simulink model "state_feedback_control_4_1_wout_velocity_eqn_2"  (R2018b)
settings: Solver=VariableStepAuto  StartTime=0.0  StopTime=10.0  RelTol=1e-3
values from neighbouring files (symbols this model uses):
  alpha = 10    [in_lab.m]
  f1 = F(1)    [in_lab.m]
  f2 = F(2)    [in_lab.m]
libraries: cstblocks x1
settings Model: Creator=pranshumalik14  LastModifiedBy=pranshumalik14

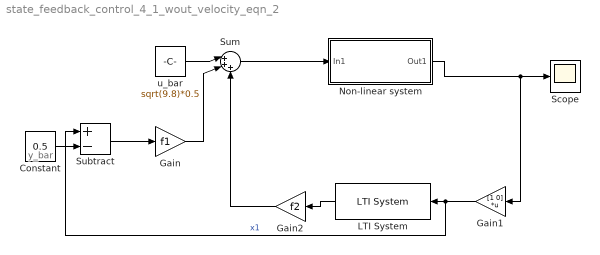
== system state_feedback_control_4_1_wout_velocity_eqn_2 ==
  note: y_bar
  Constant : Constant  Value=0.5
  Gain : Gain  Gain=f1
  Gain1 : Gain  Gain=[1 0]  Multiplication=Matrix(K*u) (u vector)
  Gain2 : Gain  Gain=f2
  LTI System : cstblocks/LTI System  sys=tf([alpha 0], [1 alpha])  IC=[]
  Non-linear system : Subsystem
  Scope : Scope
  Subtract : Sum  Inputs=+-
  Sum : Sum  Inputs=|+++
  u_bar : Constant  Value=sqrt(9.8)*0.5
  wires:
  Non-linear system/1(Out1) -> Gain1/1, Scope/1
  u_bar/1 -> Sum/1
  Sum/1 -> Non-linear system/1(In1)
  Gain/1 -> Sum/2
  Gain1/1 -> Subtract/1, LTI System/1  "x1"
  LTI System/1 -> Gain2/1
  Gain2/1 -> Sum/3
  Constant/1 -> Subtract/2
  Subtract/1 -> Gain/1

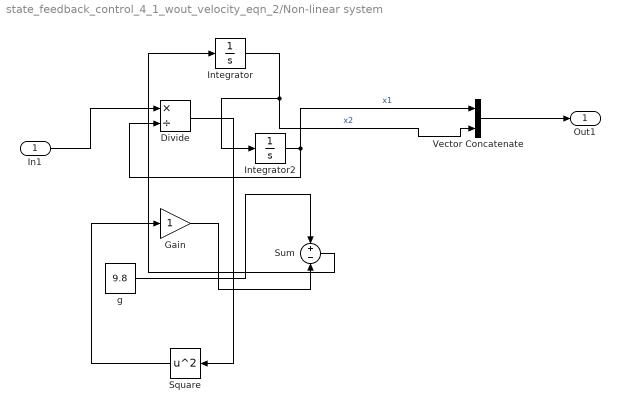
== system state_feedback_control_4_1_wout_velocity_eqn_2/Non-linear system ==
  In1 : Inport
  Divide : Product  Inputs=*/
  Gain : Gain
  Integrator : Integrator  InitialCondition=0.5
  Integrator2 : Integrator  InitialCondition=1.3
  Square : Math  Operator=square  SaturateOnIntegerOverflow=on
  Sum : Sum  Inputs=+-
  Vector Concatenate : Concatenate
  g : Constant  Value=9.8
  Out1 : Outport
  wires:
  Integrator2/1 -> Vector Concatenate/1, Divide/2  "x1"
  Integrator/1 -> Vector Concatenate/2, Integrator2/1  "x2"
  In1/1 -> Divide/1
  g/1 -> Sum/1
  Divide/1 -> Square/1
  Square/1 -> Gain/1
  Gain/1 -> Sum/2
  Sum/1 -> Integrator/1
  Vector Concatenate/1 -> Out1/1
